simulink subsystem "Enviroment"  (R2022b)
settings: Solver=VariableStepAuto  StartTime=0.0  StopTime=10.0  RelTol=1e-3
undefined symbols (not defined in the file or in its folder): environment, settings
settings Model: Creator=robertopistonenascone  LastModifiedBy=robertopistonenascone

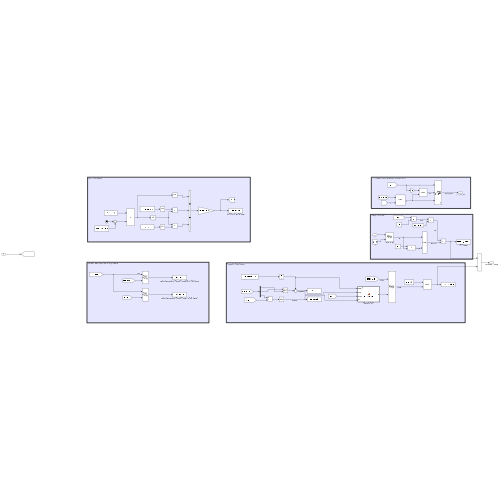
[thumbnail: Simulink's stored preview of the top-level diagram]
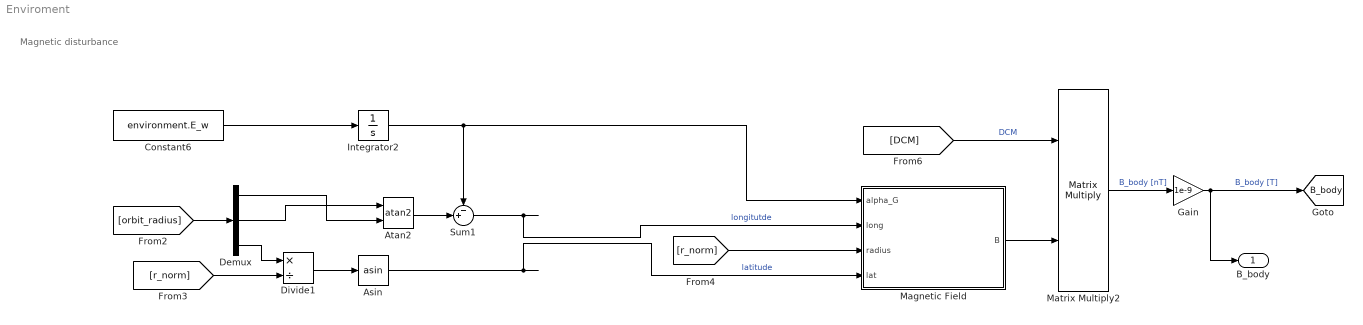
== system Enviroment ==
  note: Magnetic disturbance
  Asin : Trigonometry  Operator=asin
  Atan2 : Trigonometry  Operator=atan2
  Constant6 : Constant  Value=environment.E_w
  Demux : Demux  Outputs=3
  Divide1 : Product  Inputs=*/
  Gain : Gain  Gain=1e-9
  Integrator2 : Integrator  InitialCondition=environment.theta_G0
  Magnetic Field : MATLAB Function  TreatAsAtomicUnit=on
  Matrix Multiply2 : Product  Multiplication=Matrix(*)
  Sum1 : Sum  Inputs=-+|
  B_body : Outport
  tag scope: B_body=global
  wires:
  Atan2/1 -> Sum1/2
  Demux/2 -> Atan2/1
  Integrator2/1 -> Magnetic Field/1(alpha_G), Sum1/1
  [orbit_radius] -> Demux/1
  Constant6/1 -> Integrator2/1
  Demux/1 -> Atan2/2
  Sum1/1 -> Magnetic Field/2(long)  "longitutde"
  Asin/1 -> Magnetic Field/4(lat)  "latitude"
  [r_norm] -> Divide1/2
  Divide1/1 -> Asin/1
  Matrix Multiply2/1 -> Gain/1  "B_body [nT]"
  Magnetic Field/1(B) -> Matrix Multiply2/2
  Demux/3 -> Divide1/1
  [DCM] -> Matrix Multiply2/1  "DCM"
  [r_norm] -> Magnetic Field/3(radius)
  Gain/1 -> B_body/1, [B_body]  "B_body [T]"

== matlab function Enviroment/Magnetic Field ==
  data: alpha_G input; long input; radius input; B output; lat input; environment parameter; settings parameter
function B = magneticField(alpha_G,long,radius,lat,environment,settings)
%{  
    Return the magnetic field component in inertial reference frame

%}
theta = (pi/2-lat);     % theta is the colatitude [rad]
alpha = long + alpha_G; 

g = environment.WMM.g;
h = environment.WMM.h;
K = environment.WMM.K;
R = environment.R;
N = settings.N;

%% P-dP
% validated through the P and dP tables in "Jeremy Davis, Mathematical Modeling of Earthas Magnetic
% Field, 2004"

%%%%%%%%%%%%%%%%%%%%%%%%%%%%%%%%%%%%%%%%%%%%%%%%%%%%%%%%%%%%%%%%%%%%%%%%%%%%%%%%%%%%%%%%%%%%%%%%
% P_{(n),(m+1)}: 
% given P(a,b) -> n=a, m=b-1
% n from 1 to N
% m from 0 to N
% N order of accuracy
%%%%%%%%%%%%%%%%%%%%%%%%%%%%%%%%%%%%%%%%%%%%%%%%%%%%%%%%%%%%%%%%%%%%%%%%%%%%%%%%%%%%%%%%%%%%%%%%

P = zeros(N,N+1);
dP = zeros(N,N+1);

P_00 = 1;
dP_00 = 0;

P_01 = 0; 
dP_01 = 0;

P(1,1) = cos(theta); % n=1, m=0
dP(1,1) = -sin(theta)*P_00; 

P(1,2) = sin(theta);  % n=1, m=1
dP(1,2) = cos(theta)*P_00;

for i = 2:N % ciclo in n a partire da n=2 a n=N
    for j = 0:i % ciclo in m da m=0 a m=n
        if j == i
        P(i,j+1) = sin(theta)*P(i-1,j);
        dP(i,j+1) = sin(theta)*dP(i-1,j) + cos(theta)*P(i-1,j);
        elseif i < 3
            if j == 0 % n=2, m=0
            P(i,j+1) = cos(theta)*P(i-1,j+1) - K(i,j+1)*P_00;
            dP(i,j+1) = -sin(theta)*P(i-1,j+1) + cos(theta)*dP(i-1,j+1) ...
                - K(i,j+1)*dP_00;
            elseif j == 1 % n=2, m=1
                P(i,j+1) = cos(theta)*P(i-1,j+1) - K(i,j+1)*P_01;
                dP(i,j+1) = -sin(theta)*P(i-1,j+1) + cos(theta)*dP(i-1,j+1)...
                    - K(i,j+1)*dP_01;
            end
        else
            P(i,j+1) = cos(theta)*P(i-1,j+1) - K(i,j+1)*P(i-2,j+1);
            dP(i,j+1) = -sin(theta)*P(i-1,j+1) + cos(theta)*dP(i-1,j+1) ...
                - K(i,j+1)*dP(i-2,j+1);
        end
    end
end

%% Magnetic Field

B_r = 0;
B_th = 0;
B_phi = 0;

%indice i scorre n da 1 a N
%indice j scorre m da 0 a n

for m = 0:N
    for n = 1:N
        if m<=n
            B_r = B_r + (R/radius)^(n+2)*(n+1)*...
                ((g(n,m+1)*cos(m*long) + h(n,m+1)*sin(m*long))*P(n, m+1));
            B_th = B_th + (R/radius)^(n+2)*...
                ((g(n,m+1)*cos(m*long) + h(n,m+1)*sin(m*long))*dP(n, m+1));
            B_phi = B_phi + (R/radius)^(n+2)*...
                (m*(-g(n,m+1)*sin(m*long) + h(n,m+1)*cos(m*long))* P(n, m+1));

        end

    end
end

B_th = -B_th;
B_phi = -B_phi/sin(theta);

B_x = ( B_r*cos(lat) + B_th*sin(lat) ) * cos(alpha) - B_phi*sin(alpha);
B_y = ( B_r*cos(lat) + B_th*sin(lat) ) * sin(alpha) + B_phi*cos(alpha);
B_z = B_r*sin(lat) + B_th*cos(lat);

B = [B_x B_y B_z]';
